simulink model "modelo"  (R2023b)
settings: Solver=VariableStepAuto  StartTime=0.0  StopTime=100  FixedStep=T  RelTol=1e-3
values from neighbouring files (symbols this model uses):
  alpha_k = constantes(14)    [calculaMatrizesModelo.m]    (also in simulaModeloSimulink.m; simulaTrajetoriaSimulink.m)
  alpha_s = constantes(13)    [calculaMatrizesModelo.m]    (also in simulaModeloSimulink.m; simulaTrajetoriaSimulink.m)
  b = constantes(7)    [calculaMatrizesModelo.m]    (also in simulaModeloSimulink.m; simulaTrajetoriaSimulink.m)
  d = constantes(5)    [calculaMatrizesModelo.m]    (also in simulaModeloSimulink.m; simulaTrajetoriaSimulink.m)
  f_k = constantes(12)    [calculaMatrizesModelo.m]    (also in simulaModeloSimulink.m; simulaTrajetoriaSimulink.m)
  f_s = constantes(11)    [calculaMatrizesModelo.m]    (also in simulaModeloSimulink.m; simulaTrajetoriaSimulink.m)
  g = 9.81    [calculaMatrizesModelo.m]    (also in simulaModeloSimulink.m; simulaTrajetoriaSimulink.m)
  K_ce = constantes(8)    [calculaMatrizesModelo.m]    (also in simulaModeloSimulink.m; simulaTrajetoriaSimulink.m)
  k_i = constantes(15)    [calculaMatrizesModelo.m]    (also in simulaModeloSimulink.m; simulaTrajetoriaSimulink.m)
  k_p = constantes(16)    [calculaMatrizesModelo.m]    (also in simulaModeloSimulink.m; simulaTrajetoriaSimulink.m)
  K_t = constantes(9)    [calculaMatrizesModelo.m]    (also in simulaModeloSimulink.m; simulaTrajetoriaSimulink.m)
  L = constantes(2)    [calculaMatrizesModelo.m]    (also in simulaModeloSimulink.m; simulaTrajetoriaSimulink.m)
  m = m_c + 2*m_w    [calculaMatrizesModelo.m]    (also in simulaModeloSimulink.m; simulaTrajetoriaSimulink.m)
  m_c = constantes(3)    [calculaMatrizesModelo.m]    (also in simulaModeloSimulink.m; simulaTrajetoriaSimulink.m)
  Md = (4*I_w^2*L^2 + 2*m*I_w*L^2*R^2 + 2*I_t*I_w*R^2 + I_t*m*R^4)    [simulaModeloSimulink.m]    (also in simulaTrajetoriaSimulink.m)
  Mn1 = (m*L^2*R^2 + 4*I_w*L^2 + I_t*R^2)/(4*I_w^2*L^2 + 2*m*I_w*L^2*R^2 + 2*I_t*I_w*R^2 + I_t*m*R^4)    [simulaModeloSimulink.m]    (also in simulaTrajetoriaSimulink.m)
  Mn2 = (R^2*(- m*L^2 + I_t))    [simulaModeloSimulink.m]    (also in simulaTrajetoriaSimulink.m)
  N = constantes(6)    [calculaMatrizesModelo.m]    (also in simulaModeloSimulink.m; simulaTrajetoriaSimulink.m)
  R = 0.034    [calculaErros.m]    (also in calculaMatrizesModelo.m = constantes(1); plotTrajetoria.m = 0.175; simulaModeloSimulink.m = constantes(1); simulaTrajetoriaSimulink.m = constantes(1))
  R_a = constantes(10)    [calculaMatrizesModelo.m]    (also in simulaModeloSimulink.m; simulaTrajetoriaSimulink.m)
  T = 1e-2    (= 0.01)    [otimizaControladorOnline.m]    (also in otimizaModelo.m = tempos(2)-tempos(1); otimizaModeloOffline.m; simulaModeloSimulink.m = tempo(2)-tempo(1); simulaTrajetoria.m)
libraries: slpidlib x2
settings Model: Creator=Gabriel Sousa  LastModifiedBy=Gabriel Sousa
settings DataIOCC: SaveState=on

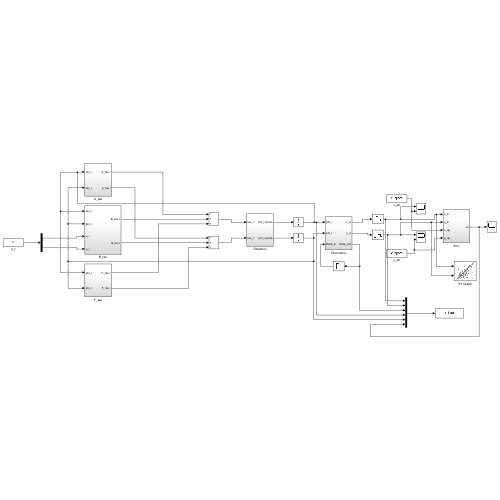
[thumbnail: Simulink's stored preview of the top-level diagram]
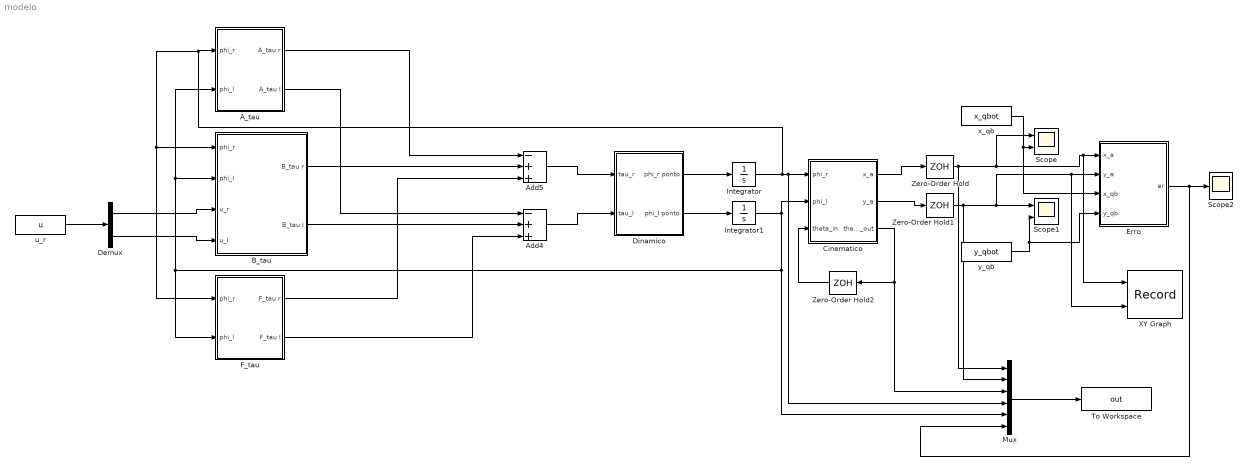
== system modelo ==
  A_tau : Subsystem
  Add4 : Sum  Inputs=-++
  Add5 : Sum  Inputs=-++
  B_tau : Subsystem
  Cinematico : Subsystem
  Demux : Demux  Outputs=2
  Dinamico : Subsystem
  Erro : Subsystem
  F_tau : Subsystem
  Integrator : Integrator
  Integrator1 : Integrator
  Mux : Mux  Inputs=6
  Scope : Scope  NumInputPorts=2
  Scope1 : Scope  NumInputPorts=2
  Scope2 : Scope
  To Workspace : ToWorkspace  VariableName=out  SaveFormat=Timeseries  SampleTime=-1
  XY Graph : Record  FileSettingsInternal="{\"entries\":[{\"content\":{\"excelSettings\":{\"content\":{},\"type\":\"Streamout.ExcelSettings\"}},\"type\":\"Streamout.FileSettingStorage\",\"uuid\":\"\"}],\"packageUris\":[\"http:\\/\\/schema.mathworks.com\\/mf0\\/streamout_blocks\\/R2020a\"],\"version\":\"1.0\"}"  Layout=[1 1]  SignalsInternal="{\"entries\":[{\"content\":{\"signals\":[{\"content\":{\"blockPath\":[],\"dimensions\":[1],\"domain\":\"\",\"lineColor\":\"#a2142f\",\"plots\":[1],\"port\":1,\"sid\":[\"\"],\"signalID\":687,\"signalName\":\"Zero-Order\\nHold\"},\"type\":\"RecordBlkView.Signal\",\"uuid\":\"\"},{\"content\":{\"blockPath\":[],\"dimensions\":[1],\"domain\":\"\",\"lineColor\":\"#139fff\",\"plots\":[1],\"port\":2,\"sid\":[\"\"],\"signalID\":691,\"signalName\":\"Zero-Order\\nHold1\"},\"type\":\"RecordBlkView.Signal\",\"uuid\":\"\"}]},\"type\":\"RecordBlkView.InputSignals\",\"uuid\":\"\"}],\"packageUris\":[\"http:\\/\\/schema.mathworks.com\\/mf0\\/streamout_blocks\\/R2020a\"],\"version\":\"1.0\"}"  VisualizationBindings="{\"xyplotplugin\":{\"info\":[{\"series\":[{\"bindingParametersList\":[{\"parameter\":\"X-Axis\",\"signalID\":687,\"signalName\":\"Zero-Order\\nHold\"},{\"parameter\":\"Y-Axis\",\"signalID\":691,\"signalName\":\"Zero-Order\\nHold1\"}],\"seriesID\":25790}],\"subplotID\":1}]}}"  CompatibilityTag=XY
  Zero-Order Hold : ZeroOrderHold  SampleTime=0.01
  Zero-Order Hold1 : ZeroOrderHold  SampleTime=0.01
  Zero-Order Hold2 : ZeroOrderHold  SampleTime=0.01
  u_r : FromWorkspace  VariableName=u  SampleTime=T
  x_qb : FromWorkspace  VariableName=x_qbot  SampleTime=T
  y_qb : FromWorkspace  VariableName=y_qbot  SampleTime=T
  wires:
  Demux/2 -> B_tau/4(u_l)
  A_tau/1(A_tau r) -> Add5/1
  B_tau/1(B_tau r) -> Add5/2
  F_tau/1(F_tau r) -> Add5/3
  A_tau/2(A_tau l) -> Add4/1
  B_tau/2(B_tau l) -> Add4/2
  F_tau/2(F_tau l) -> Add4/3
  Add5/1 -> Dinamico/1(tau_r)
  Add4/1 -> Dinamico/2(tau_l)
  Dinamico/1(phi_r ponto) -> Integrator/1
  Dinamico/2(phi_l ponto) -> Integrator1/1
  Zero-Order Hold/1 -> Scope/1, XY Graph/1, Erro/1(x_a), Mux/1
  Zero-Order Hold1/1 -> XY Graph/2, Erro/2(y_a), Scope1/1, Mux/2
  y_qb/1 -> Erro/4(y_qb), Scope1/2
  x_qb/1 -> Erro/3(x_qb), Scope/2
  Erro/1(er) -> Mux/6, Scope2/1
  Cinematico/1(x_a) -> Zero-Order Hold/1
  Cinematico/2(y_a) -> Zero-Order Hold1/1
  Integrator/1 -> Cinematico/1(phi_r), Mux/4, F_tau/1(phi_r), B_tau/1(phi_r), A_tau/1(phi_r)
  Integrator1/1 -> Mux/5, B_tau/2(phi_l), A_tau/2(phi_l), F_tau/2(phi_l), Cinematico/2(phi_l)
  Cinematico/3(theta_out) -> Mux/3, Zero-Order Hold2/1
  Zero-Order Hold2/1 -> Cinematico/3(theta_in)
  Mux/1 -> To Workspace/1
  Demux/1 -> B_tau/3(u_r)
  u_r/1 -> Demux/1

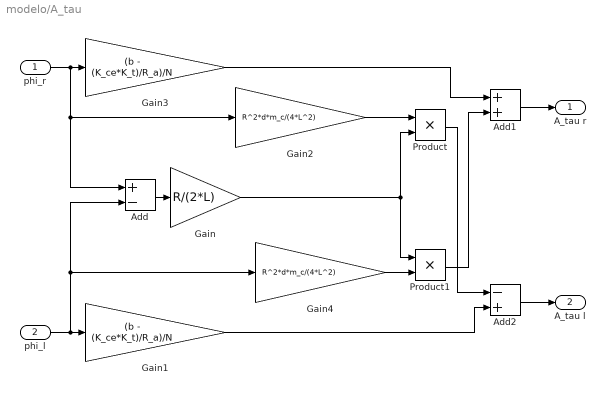
== system modelo/A_tau ==
  phi_r : Inport
  phi_l : Inport  Port=2
  Add : Sum  Inputs=+-
  Add1 : Sum
  Add2 : Sum  Inputs=-+
  Gain : Gain  Gain=R/(2*L)
  Gain1 : Gain  Gain=(b - (K_ce*K_t)/R_a)/N
  Gain2 : Gain  Gain=R^2*d*m_c/(4*L^2)
  Gain3 : Gain  Gain=(b - (K_ce*K_t)/R_a)/N
  Gain4 : Gain  Gain=R^2*d*m_c/(4*L^2)
  Product : Product
  Product1 : Product
  A_tau r : Outport
  A_tau l : Outport  Port=2
  wires:
  phi_r/1 -> Gain2/1, Add/1, Gain3/1
  Gain3/1 -> Add1/1
  Gain1/1 -> Add2/2
  phi_l/1 -> Gain1/1, Gain4/1, Add/2
  Add/1 -> Gain/1
  Gain4/1 -> Product1/2
  Gain/1 -> Product/2, Product1/1
  Gain2/1 -> Product/1
  Product1/1 -> Add1/2
  Product/1 -> Add2/1
  Add2/1 -> A_tau l/1
  Add1/1 -> A_tau r/1

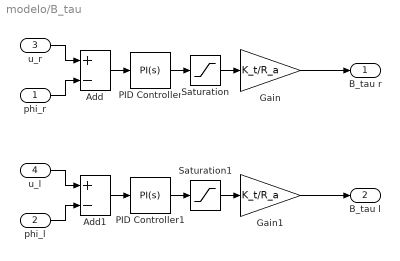
== system modelo/B_tau ==
  phi_r : Inport
  phi_l : Inport  Port=2
  u_r : Inport  Port=3
  u_l : Inport  Port=4
  Add : Sum  Inputs=+-
  Add1 : Sum  Inputs=+-
  Gain : Gain  Gain=K_t/R_a
  Gain1 : Gain  Gain=K_t/R_a
  PID Controller : slpidlib/PID Controller  Controller=PI  Form=Ideal  TimeDomain=Continuous-time  UseExternalTs=off  SampleTime=-1  IntegratorMethod=Forward Euler  FilterMethod=Forward Euler  ControllerParametersSource=internal  P=k_p  I=k_i  UseKiTs=off  D=0  N=100  UseFilter=on  TunerSelectOption=Transfer Function Based (PID Tuner App)  InitialConditionSource=internal  InitialConditionForIntegrator=0  InitialConditionForFilter=0  DifferentiatorICPrevScaledInput=0  ExternalReset=none  TrackingMode=off  Kt=1  LimitOutput=off  SatLimitsSource=internal  UpperSaturationLimit=inf  LowerSaturationLimit=-inf  LinearizeAsGain=on  AntiWindupMode=none  Kb=1  LimitIntegrator=off  UpperIntegratorSaturationLimit=inf  LowerIntegratorSaturationLimit=-inf  POutMin=[]  POutMax=[]  IOutMin=[]  IOutMax=[]  DOutMin=[]  DOutMax=[]  NOutMin=[]  NOutMax=[]  SumOutMin=[]  SumOutMax=[]  SaturationOutMin=[]  SaturationOutMax=[]  PParamMin=[]  PParamMax=[]  IParamMin=[]  IParamMax=[]  DParamMin=[]  DParamMax=[]  NParamMin=[]  NParamMax=[]  KbParamMin=[]  KbParamMax=[]  KtParamMin=[]  KtParamMax=[]  KbOutMin=[]  KbOutMax=[]  KtOutMin=[]  KtOutMax=[]  IntegratorOutMin=[]  IntegratorOutMax=[]  FilterOutMin=[]  FilterOutMax=[]  SumI1OutMin=[]  SumI1OutMax=[]  SumI2OutMin=[]  SumI2OutMax=[]  SumI3OutMin=[]  SumI3OutMax=[]  SumI4OutMin=[]  SumI4OutMax=[]  SumDOutMin=[]  SumDOutMax=[]  DifferentiatorOutMin=[]  DifferentiatorOutMax=[]  FilterDiffOutCoefMin=[]  FilterDiffOutCoefMax=[]  ReciprocalOutMin=[]  ReciprocalOutMax=[]  SumDenOutMin=[]  SumDenOutMax=[]  SumNumOutMin=[]  SumNumOutMax=[]  DivideOutMin=[]  DivideOutMax=[]  UdiffTsProdOutMin=[]  UdiffTsProdOutMax=[]  NTsProdOutMin=[]  NTsProdOutMax=[]  UintegralTsProdOutMin=[]  UintegralTsProdOutMax=[]  UngainTsProdOutMin=[]  UngainTsProdOutMax=[]  ClampingZeroOutDataTypeStr=Inherit: Inherit via back propagation  ClampingZeroOutMin=[]  ClampingZeroOutMax=[]  FilterDenConstantOutDataTypeStr=Inherit: Inherit via back propagation  FilterDenConstantOutMin=[]  FilterDenConstantOutMax=[]  PCopyOutDataTypeStr=Inherit: Inherit via back propagation  PCopyOutMin=[]  PCopyOutMax=[]  NCopyOutDataTypeStr=Inherit: Inherit via back propagation  NCopyOutMin=[]  NCopyOutMax=[]  IntegratorContinuousStateAttributes=''  IntegratorStateMustResolveToSignalObject=off  IntegratorRTWStateStorageClass=Auto  FilterContinuousStateAttributes=''  FilterStateMustResolveToSignalObject=off  FilterRTWStateStorageClass=Auto  ParallelPVariant=Passthrough  IdealPVariant=InternalParameters  IVariant=InternalParameters  DVariant=Disabled  IntegratorVariant=Continuous  SatVariant=Disabled  AWVariant=Passthrough  PCopyVariant=Disabled  TRVariant=Disabled  FdbkBlocksVariant=Forward  IdealPFdbkVariant=Disabled  SatFdbkVariant=Disabled  DerivativeFilterVariant=Disabled  NVariant=Disabled  NCopyVariant=Disabled_SignalSpec  FilterICVariant=Disabled  IntegratorICVariant=InternalICs  ExternalResetVariant=Disabled  TRSumVariant=Passthrough  SumFdbkVariant=Disabled  SumVariant=Sum_PI  TsampFilterVariant=InternalTs  TsampNgainVariant=Passthrough  TsampIntegralVariant=Disabled_SignalSpec  ExternalSaturationOutDataTypeStr=Inherit: Same as second input
  PID Controller1 : slpidlib/PID Controller  Controller=PI  Form=Ideal  TimeDomain=Continuous-time  UseExternalTs=off  SampleTime=-1  IntegratorMethod=Forward Euler  FilterMethod=Forward Euler  ControllerParametersSource=internal  P=k_p  I=k_i  UseKiTs=off  D=0  N=100  UseFilter=on  TunerSelectOption=Transfer Function Based (PID Tuner App)  InitialConditionSource=internal  InitialConditionForIntegrator=0  InitialConditionForFilter=0  DifferentiatorICPrevScaledInput=0  ExternalReset=none  TrackingMode=off  Kt=1  LimitOutput=off  SatLimitsSource=internal  UpperSaturationLimit=inf  LowerSaturationLimit=-inf  LinearizeAsGain=on  AntiWindupMode=none  Kb=1  LimitIntegrator=off  UpperIntegratorSaturationLimit=inf  LowerIntegratorSaturationLimit=-inf  POutMin=[]  POutMax=[]  IOutMin=[]  IOutMax=[]  DOutMin=[]  DOutMax=[]  NOutMin=[]  NOutMax=[]  SumOutMin=[]  SumOutMax=[]  SaturationOutMin=[]  SaturationOutMax=[]  PParamMin=[]  PParamMax=[]  IParamMin=[]  IParamMax=[]  DParamMin=[]  DParamMax=[]  NParamMin=[]  NParamMax=[]  KbParamMin=[]  KbParamMax=[]  KtParamMin=[]  KtParamMax=[]  KbOutMin=[]  KbOutMax=[]  KtOutMin=[]  KtOutMax=[]  IntegratorOutMin=[]  IntegratorOutMax=[]  FilterOutMin=[]  FilterOutMax=[]  SumI1OutMin=[]  SumI1OutMax=[]  SumI2OutMin=[]  SumI2OutMax=[]  SumI3OutMin=[]  SumI3OutMax=[]  SumI4OutMin=[]  SumI4OutMax=[]  SumDOutMin=[]  SumDOutMax=[]  DifferentiatorOutMin=[]  DifferentiatorOutMax=[]  FilterDiffOutCoefMin=[]  FilterDiffOutCoefMax=[]  ReciprocalOutMin=[]  ReciprocalOutMax=[]  SumDenOutMin=[]  SumDenOutMax=[]  SumNumOutMin=[]  SumNumOutMax=[]  DivideOutMin=[]  DivideOutMax=[]  UdiffTsProdOutMin=[]  UdiffTsProdOutMax=[]  NTsProdOutMin=[]  NTsProdOutMax=[]  UintegralTsProdOutMin=[]  UintegralTsProdOutMax=[]  UngainTsProdOutMin=[]  UngainTsProdOutMax=[]  ClampingZeroOutDataTypeStr=Inherit: Inherit via back propagation  ClampingZeroOutMin=[]  ClampingZeroOutMax=[]  FilterDenConstantOutDataTypeStr=Inherit: Inherit via back propagation  FilterDenConstantOutMin=[]  FilterDenConstantOutMax=[]  PCopyOutDataTypeStr=Inherit: Inherit via back propagation  PCopyOutMin=[]  PCopyOutMax=[]  NCopyOutDataTypeStr=Inherit: Inherit via back propagation  NCopyOutMin=[]  NCopyOutMax=[]  IntegratorContinuousStateAttributes=''  IntegratorStateMustResolveToSignalObject=off  IntegratorRTWStateStorageClass=Auto  FilterContinuousStateAttributes=''  FilterStateMustResolveToSignalObject=off  FilterRTWStateStorageClass=Auto  ParallelPVariant=Passthrough  IdealPVariant=InternalParameters  IVariant=InternalParameters  DVariant=Disabled  IntegratorVariant=Continuous  SatVariant=Disabled  AWVariant=Passthrough  PCopyVariant=Disabled  TRVariant=Disabled  FdbkBlocksVariant=Forward  IdealPFdbkVariant=Disabled  SatFdbkVariant=Disabled  DerivativeFilterVariant=Disabled  NVariant=Disabled  NCopyVariant=Disabled_SignalSpec  FilterICVariant=Disabled  IntegratorICVariant=InternalICs  ExternalResetVariant=Disabled  TRSumVariant=Passthrough  SumFdbkVariant=Disabled  SumVariant=Sum_PI  TsampFilterVariant=InternalTs  TsampNgainVariant=Passthrough  TsampIntegralVariant=Disabled_SignalSpec  ExternalSaturationOutDataTypeStr=Inherit: Same as second input
  Saturation : Saturate  UpperLimit=12  LowerLimit=-12
  Saturation1 : Saturate  UpperLimit=12  LowerLimit=-12
  B_tau r : Outport
  B_tau l : Outport  Port=2
  wires:
  Gain/1 -> B_tau r/1
  Add/1 -> PID Controller/1
  PID Controller/1 -> Saturation/1
  Saturation/1 -> Gain/1
  phi_r/1 -> Add/2
  Saturation1/1 -> Gain1/1
  Add1/1 -> PID Controller1/1
  phi_l/1 -> Add1/2
  PID Controller1/1 -> Saturation1/1
  Gain1/1 -> B_tau l/1
  u_r/1 -> Add/1
  u_l/1 -> Add1/1

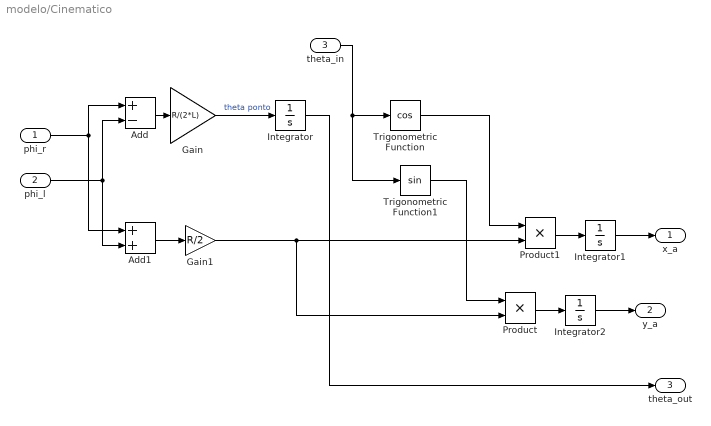
== system modelo/Cinematico ==
  phi_r : Inport
  phi_l : Inport  Port=2
  theta_in : Inport  Port=3
  Add : Sum  Inputs=+-
  Add1 : Sum
  Gain : Gain  Gain=R/(2*L)
  Gain1 : Gain  Gain=R/2
  Integrator : Integrator
  Integrator1 : Integrator
  Integrator2 : Integrator
  Product : Product
  Product1 : Product
  Trigonometric Function : Trigonometry  Operator=cos
  Trigonometric Function1 : Trigonometry
  x_a : Outport  VectorParamsAs1DForOutWhenUnconnected=off
  y_a : Outport  Port=2  VectorParamsAs1DForOutWhenUnconnected=off
  theta_out : Outport  Port=3  VectorParamsAs1DForOutWhenUnconnected=off
  wires:
  phi_r/1 -> Add/1, Add1/1
  phi_l/1 -> Add/2, Add1/2
  Add/1 -> Gain/1
  Gain/1 -> Integrator/1  "theta ponto"
  Add1/1 -> Gain1/1
  Trigonometric Function/1 -> Product1/1
  Trigonometric Function1/1 -> Product/1
  Product/1 -> Integrator2/1
  Product1/1 -> Integrator1/1
  Integrator1/1 -> x_a/1
  Integrator2/1 -> y_a/1
  Gain1/1 -> Product1/2, Product/2
  theta_in/1 -> Trigonometric Function1/1, Trigonometric Function/1
  Integrator/1 -> theta_out/1

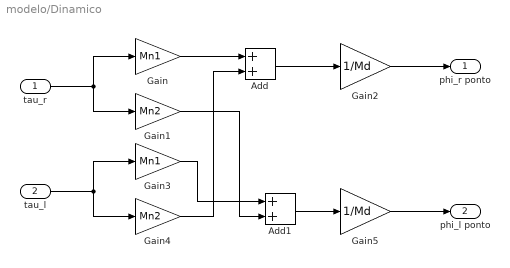
== system modelo/Dinamico ==
  tau_r : Inport
  tau_l : Inport  Port=2
  Add : Sum
  Add1 : Sum
  Gain : Gain  Gain=Mn1
  Gain1 : Gain  Gain=Mn2
  Gain2 : Gain  Gain=1/Md
  Gain3 : Gain  Gain=Mn1
  Gain4 : Gain  Gain=Mn2
  Gain5 : Gain  Gain=1/Md
  phi_r ponto : Outport  VectorParamsAs1DForOutWhenUnconnected=off
  phi_l ponto : Outport  Port=2  VectorParamsAs1DForOutWhenUnconnected=off
  wires:
  tau_r/1 -> Gain/1, Gain1/1
  tau_l/1 -> Gain3/1, Gain4/1
  Gain5/1 -> phi_l ponto/1
  Gain2/1 -> phi_r ponto/1
  Gain/1 -> Add/1
  Gain4/1 -> Add/2
  Gain3/1 -> Add1/1
  Gain1/1 -> Add1/2
  Add1/1 -> Gain5/1
  Add/1 -> Gain2/1

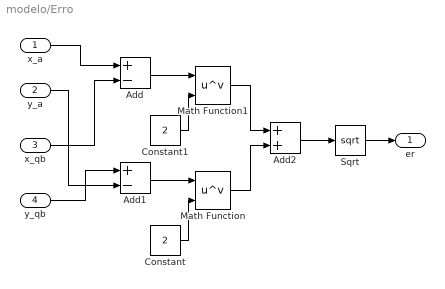
== system modelo/Erro ==
  x_a : Inport
  y_a : Inport  Port=2
  x_qb : Inport  Port=3
  y_qb : Inport  Port=4
  Add : Sum  Inputs=+-
  Add1 : Sum  Inputs=+-
  Add2 : Sum
  Constant : Constant  Value=2
  Constant1 : Constant  Value=2
  Math Function : Math  Operator=pow
  Math Function1 : Math  Operator=pow
  Sqrt : Sqrt
  er : Outport
  wires:
  x_a/1 -> Add/1
  x_qb/1 -> Add/2
  y_qb/1 -> Add1/1
  y_a/1 -> Add1/2
  Add1/1 -> Math Function/1
  Add/1 -> Math Function1/1
  Constant1/1 -> Math Function1/2
  Constant/1 -> Math Function/2
  Math Function/1 -> Add2/2
  Math Function1/1 -> Add2/1
  Add2/1 -> Sqrt/1
  Sqrt/1 -> er/1

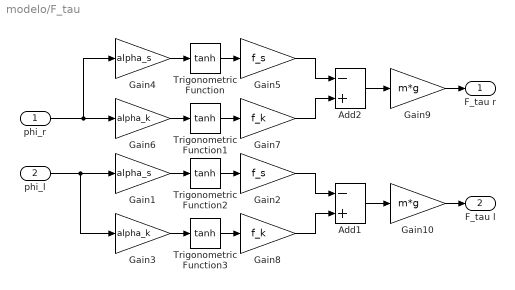
== system modelo/F_tau ==
  phi_r : Inport
  phi_l : Inport  Port=2
  Add1 : Sum  Inputs=-+
  Add2 : Sum  Inputs=-+
  Gain1 : Gain  Gain=alpha_s
  Gain10 : Gain  Gain=m*g
  Gain2 : Gain  Gain=f_s
  Gain3 : Gain  Gain=alpha_k
  Gain4 : Gain  Gain=alpha_s
  Gain5 : Gain  Gain=f_s
  Gain6 : Gain  Gain=alpha_k
  Gain7 : Gain  Gain=f_k
  Gain8 : Gain  Gain=f_k
  Gain9 : Gain  Gain=m*g
  Trigonometric Function{,1..3} (4 alike) : Trigonometry  Operator=tanh
  F_tau r : Outport
  F_tau l : Outport  Port=2
  wires:
  Gain5/1 -> Add2/1
  Trigonometric Function/1 -> Gain5/1
  Gain4/1 -> Trigonometric Function/1
  Gain6/1 -> Trigonometric Function1/1
  Gain7/1 -> Add2/2
  Trigonometric Function1/1 -> Gain7/1
  phi_r/1 -> Gain4/1, Gain6/1
  Trigonometric Function3/1 -> Gain8/1
  Gain1/1 -> Trigonometric Function2/1
  Gain2/1 -> Add1/1
  Gain8/1 -> Add1/2
  Trigonometric Function2/1 -> Gain2/1
  Gain3/1 -> Trigonometric Function3/1
  phi_l/1 -> Gain3/1, Gain1/1
  Add2/1 -> Gain9/1
  Add1/1 -> Gain10/1
  Gain9/1 -> F_tau r/1
  Gain10/1 -> F_tau l/1
